simulink model "realtime"  (R2024b)
settings: Solver=ode5  StartTime=0.0  StopTime=45  FixedStep=0.001  RelTol=1e-3
InitFcn:
  | Init
values from neighbouring files (symbols this model uses):
  Beq = 1.223604206496999e-06    (= 1.2236042065e-06)    [DesignPart567.m]    (also in DesignPart9Sine.m; DesignPart9Step.m; Init.m; Real_time_parameter_estimation.m = (data.Beq_hat_pos + data.Beq_hat_neg)/2)
  degs2rpm = 60/360    (= 0.166666666667)    [Init.m]
  delta_est = 1/sqrt(2)    [DesignPart9Step.m]    (also in Init.m)
  Kd = Kp * Td    [Init.m]
  Ki = Kp / Ti    [Init.m]
  Kp = deltak * cos(deltaphi)    [Init.m]
  rpm2degs = 360/60    (= 6)    [Init.m]
  rpm2rads = 2*pi/60    (= 0.10471975512)    [Init.m]
  tau_sf = (abs(data.tau_sf_pos)+abs(data.tau_sf_neg))/2    [Real_time_parameter_estimation.m]    (also in real-time-estimation.mat = 0.0046178193958)
  tl = 1/(3*wgc)    [Init.m]
  wc = 2*pi*50    (= 314.159265359)    [DesignPart9Step.m]    (also in Init.m; State_space_1324.m)
undefined symbols (not defined in the file or in its folder): gbox, mld, mot, National_Instruments, PCI, sens
libraries: sldrtlib x3, simulink x2, SignalEditorBlockLib x1
settings Model: SimulationMode=external  ExtModeTrigDuration=1000001  Creator=galeazzolu  LastModifiedBy=galeazzolu
settings DataIOCC: ReturnWorkspaceOutputs=off
settings HardwareCC: ProdBitPerLong=64  ProdHWDeviceType=Intel->x86-64 (Linux 64)
settings RTWCC: Description=Simulink Desktop Real-Time  SystemTargetFile=sldrt.tlc  TemplateMakefile=sldrt.tmf  RTWCompilerOptimization=on
settings CodeAppCC: MaxIdLength=95
settings SimulinkDesktopRealTimeCC: TargetLibSuffix=_sldrt.a  TargetPreCompLibLocation=C:\Program Files\MATLAB\R2024b\toolbox\sldrt\lib\win64  ParMdlRefBuildCompliant=on

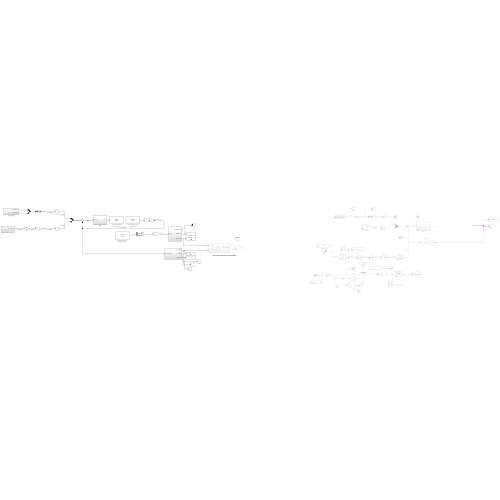
[thumbnail: Simulink's stored preview of the top-level diagram]
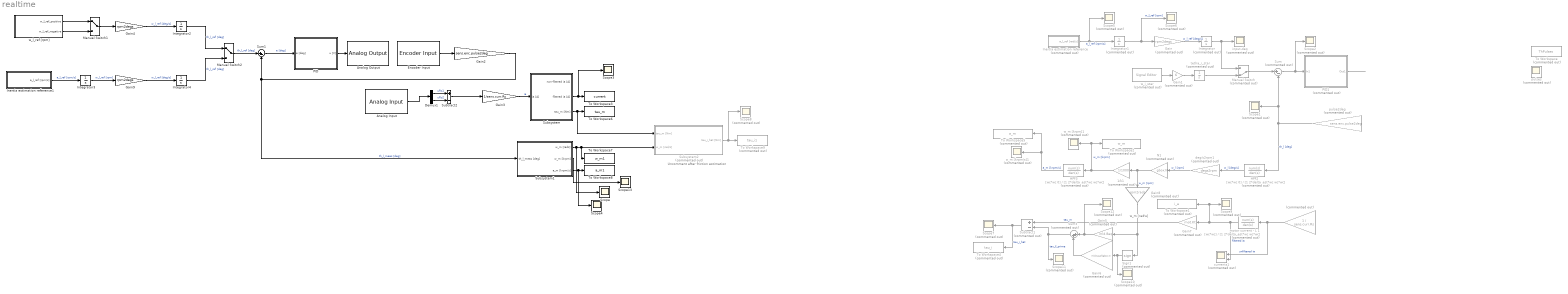
== system realtime ==
  note: w_m [rad\s]
  note: Uncomment after friction estimation
  " " : Gain  Commented=on  Gain=1 / sens.curr.Rs
  1/k1 : Gain  Commented=on  Gain=1/1000
  Analog Input : sldrtlib/Analog Input  SampleTime=-1  MaxMissedTicks=10  ShowMissedTicks=off  YieldWhenWaiting=off  DrvName=National_Instruments/PCI-6221  DrvAddress=4294967295  DrvOptions=[0 0 0 2 0]  Channels=[1,2]  RangeMode=1  VoltRange=1  DataType=1
      settings: AttributesFormatString=National Instruments\nPCI-6221 [auto]
  Analog Output : sldrtlib/Analog Output  SampleTime=-1  MaxMissedTicks=10  ShowMissedTicks=off  YieldWhenWaiting=off  DrvName=National_Instruments/PCI-6221  DrvAddress=4294967295  DrvOptions=[0 0 0 2 0]  Channels=1  RangeMode=1  VoltRange=1  InitialValue=0  FinalValue=0
      settings: AttributesFormatString=National Instruments\nPCI-6221 [auto]
  Demux1 : Demux  Outputs=2
  Encoder Input : sldrtlib/Encoder Input  SampleTime=-1  MaxMissedTicks=10  ShowMissedTicks=off  YieldWhenWaiting=off  DrvName=National_Instruments/PCI-6221  DrvAddress=4294967295  DrvOptions=[0 0 0 2 0]  Channels=1  QuadMode=3  IndexPulse=1  InputFilter=Inf  DataType=1
      settings: AttributesFormatString=National Instruments\nPCI-6221 [auto]
  Gain : Gain  Commented=on  Gain=rpm2degs
  Gain1 : Gain  Commented=on  Gain=6
  Gain2 : Gain  Gain=sens.enc.pulse2deg
  Gain3 : Gain  Gain=1/sens.curr.Rs
  Gain4 : Gain  Gain=rpm2degs
  Gain5 : Gain  Commented=on  Gain=mld.Beq
  Gain6 : Gain  Commented=on  Gain=mld.tausf/gbox.N
  Gain7 : Gain  Commented=on  Gain=mot.Kt
  Gain8 : Gain  Commented=on  Gain=rpm2rads
  Gain9 : Gain  Gain=rpm2degs
  HPF2 : TransferFcn  Commented=on  Numerator=[wc*wc 0]  Denominator=[1 2*delta_est*wc wc*wc]
  HPF3 : TransferFcn  Commented=on  Numerator=[wc*wc 0]  Denominator=[1 2*delta_est*wc wc*wc]
  Inertia estimation reference : Subsystem  Commented=on
  Inertia estimation reference1 : Subsystem
  Integrator : Integrator  Commented=on
  Integrator1 : Integrator  Commented=on
  Integrator2 : Integrator
  Integrator3 : Integrator
  Integrator4 : Integrator
  Manual Switch : ManualSwitch  Commented=on  CurrentSetting=0
  Manual Switch1 : ManualSwitch
  Manual Switch2 : ManualSwitch
  N1 : Gain  Commented=on  Gain=gbox.N
  PID : Subsystem
  PID1 : Subsystem  Commented=on
  Scope{,3..4,13} (4 alike) : Scope
  Scope{1..2,5..12} (10 alike) : Scope  Commented=on
  Sign1 : Signum  Commented=on  ZeroCross=off
  Subsystem : Subsystem
  Subsystem1 : Subsystem
  Subsystem2 : Subsystem  Commented=on
  Subtract1 : Sum  Commented=on  Inputs=+-
  Subtract2 : Sum  Inputs=+-
  Sum : Sum  Commented=on  Inputs=|+-
  Sum1 : Sum  Inputs=|+-
  Sum3 : Sum  Commented=on  Inputs=|++
  To Workspace : ToWorkspace  Commented=on  VariableName=ThPulses  SaveFormat=Structure With Time  SampleTime=-1
  To Workspace1 : ToWorkspace  Commented=on  VariableName=i_a  SaveFormat=Structure With Time  SampleTime=-1
  To Workspace2 : ToWorkspace  Commented=on  VariableName=w_m  SaveFormat=Structure With Time  SampleTime=-1
  To Workspace3 : ToWorkspace  VariableName=current  SaveFormat=Structure With Time  SampleTime=-1
  To Workspace4 : ToWorkspace  Commented=on  VariableName=tau_i  SaveFormat=Structure With Time  SampleTime=-1
  To Workspace5 : ToWorkspace  Commented=on  VariableName=a_m  SaveFormat=Structure With Time  SampleTime=-1
  To Workspace6 : ToWorkspace  VariableName=tau_m  SaveFormat=Structure With Time  SampleTime=-1
  To Workspace7 : ToWorkspace  VariableName=w_m1  SaveFormat=Structure With Time  SampleTime=-1
  To Workspace8 : ToWorkspace  VariableName=a_m1  SaveFormat=Structure With Time  SampleTime=-1
  To Workspace9 : ToWorkspace  Commented=on  VariableName=tau_i1  SaveFormat=Structure With Time  SampleTime=-1
  a_m [krpm/s]1 : Scope  Commented=on
  currents1 : Scope  Commented=on  NumInputPorts=2
  deg/s2rpm1 : Gain  Commented=on  Gain=degs2rpm
  input-deg : Scope  Commented=on
  motor current - L 1 : TransferFcn  Commented=on  Numerator=[wc*wc]  Denominator=[1 2*delta_est*wc wc*wc]
  pulse2deg : Gain  Commented=on  Gain=sens.enc.pulse2deg
  pulses : Scope  Commented=on
  tetha_i_star : Integrator  Commented=on
  w_i_star : SignalEditorBlockLib/Signal Editor  Commented=on  FileName=untitled.mat  ActiveScenario=Scenario  ActiveSignal=Signal 1  IsBus=off  OutputBusObjectStr=Bus: BusObject  SampleTime=0  Interpolate=off  ZeroCross=off  OutputAfterFinalValue=Setting to zero  Unit=inherit  PreserveSignalName=on  ApplySigPropsToAllScenarios=on  ApplySigPropsToAllSignals=off
  w_l_ref [rpm] : Subsystem
  w_m [krpm]1 : Scope  Commented=on
  wires:
  N1/1 -> Gain8/1, 1/k1/1  "w_m [rpm]"
  pulse2deg/1 -> HPF2/1, Sum/2, Scope1/1  "th_l [deg]"
  Sum3/1 -> Subtract1/2, Scope11/1  "tau_f_prime"
  motor current - L 1/1 -> To Workspace1/1, Scope9/1, Gain7/1, currents1/2  "filtered ia"
  Gain/1 -> Integrator/1  "w_l_ref [deg/s]"
  Subtract1/1 -> To Workspace4/1, Scope7/1  "tau_i_hat"
  Gain7/1 -> Subtract1/1  "tau_m"
  HPF2/1 -> deg/s2rpm1/1  "w_l [deg/s]"
  Integrator/1 -> Manual Switch/1, input-deg/1
  ? -> pulses/1, pulse2deg/1, To Workspace/1
  Inertia estimation reference/1(a_l_ref [rad/s]) -> Scope5/1, Integrator1/1  "a_l_ref [rpm/s]"
  Manual Switch/1 -> Sum/1
  Sign1/1 -> Scope10/1, Gain6/1
  deg/s2rpm1/1 -> N1/1  "w_l [rpm]"
  1/k1/1 -> HPF3/1, To Workspace2/1, w_m [krpm]1/1  "w_m [krpm]"
  HPF3/1 -> a_m [krpm/s]1/1, To Workspace5/1  "a_m [krpm/s]"
  PID1/1(Out1) -> ?
  Gain5/1 -> Sum3/1, Scope12/1
  Gain8/1 -> Sign1/1, Gain5/1
  Integrator1/1 -> Scope6/1, Gain/1  "w_l_ref [rpm]"
  Gain6/1 -> Sum3/2
  " "/1 -> currents1/1, motor current - L 1/1  "unfiltered ia"
  Sum/1 -> Scope2/1, PID1/1(In1)
  Gain1/1 -> tetha_i_star/1
  w_i_star/1 -> Gain1/1
  tetha_i_star/1 -> Manual Switch/2
  Subtract2/1 -> Gain3/1
  Manual Switch1/1 -> Gain4/1
  Integrator4/1 -> Manual Switch2/2  "th_l_ref [deg]"
  Inertia estimation reference1/1(a_l_ref [rpm/s]) -> Integrator3/1  "a_l_ref [rpm/s]"
  Encoder Input/1 -> Gain2/1
  Sum1/1 -> PID/1(e [deg])  "e [deg]"
  Gain2/1 -> Subsystem1/1(th_l_meas [deg]), Sum1/2  "th_l_meas [deg]"
  Demux1/2 -> Subtract2/2  "uRs2"
  Gain4/1 -> Integrator2/1  "w_l_ref [deg/s]"
  Gain3/1 -> Subsystem/1(ia [A])  "ia"
  Subsystem2/1(tau_i_hat [Nm]) -> Scope8/1, To Workspace9/1
  w_l_ref [rpm]/1(w_l_ref_positive) -> Manual Switch1/1
  Subsystem/3(tau_m [Nm]) -> Subsystem2/1(tau_m [Nm]), To Workspace6/1
  Integrator2/1 -> Manual Switch2/1  "th_l_ref [deg]"
  Subsystem/2(filtered ia [A]) -> Scope3/1, To Workspace3/1
  Analog Input/1 -> Demux1/1
  Integrator3/1 -> Gain9/1  "w_l_ref [rpm]"
  Subsystem1/1(w_m [rads]) -> Subsystem2/2(w_m [rad/s]), To Workspace7/1, Scope/1
  w_l_ref [rpm]/2(w_l_ref_negative) -> Manual Switch1/2
  PID/1(u [V]) -> Analog Output/1
  Subsystem1/2(w_m [krpm]) -> Scope13/1
  Manual Switch2/1 -> Sum1/1  "th_l_ref [deg]"
  Gain9/1 -> Integrator4/1  "w_l_ref [deg/s]"
  Demux1/1 -> Subtract2/1  "uRs1"
  Subsystem1/3(a_m [krpm/s]) -> Scope4/1, To Workspace8/1

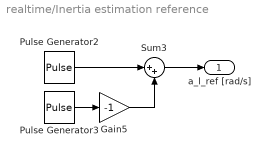
== system realtime/Inertia estimation reference ==
  Gain5 : Gain  Gain=-1
  Pulse Generator2 : DiscretePulseGenerator  PulseType=Time based  Amplitude=450  PulseWidth=50
  Pulse Generator3 : DiscretePulseGenerator  PulseType=Time based  Amplitude=450  PulseWidth=50  PhaseDelay=1
  Sum3 : Sum  Inputs=|++
  a_l_ref [rad/s] : Outport
  wires:
  Pulse Generator3/1 -> Gain5/1
  Pulse Generator2/1 -> Sum3/1
  Gain5/1 -> Sum3/2
  Sum3/1 -> a_l_ref [rad/s]/1

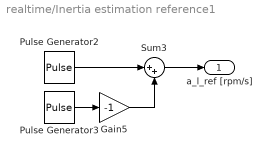
== system realtime/Inertia estimation reference1 ==
  Gain5 : Gain  Gain=-1
  Pulse Generator2 : DiscretePulseGenerator  PulseType=Time based  Amplitude=450  PulseWidth=50
  Pulse Generator3 : DiscretePulseGenerator  PulseType=Time based  Amplitude=450  PulseWidth=50  PhaseDelay=1
  Sum3 : Sum  Inputs=|++
  a_l_ref [rpm/s] : Outport
  wires:
  Pulse Generator3/1 -> Gain5/1
  Pulse Generator2/1 -> Sum3/1
  Gain5/1 -> Sum3/2
  Sum3/1 -> a_l_ref [rpm/s]/1

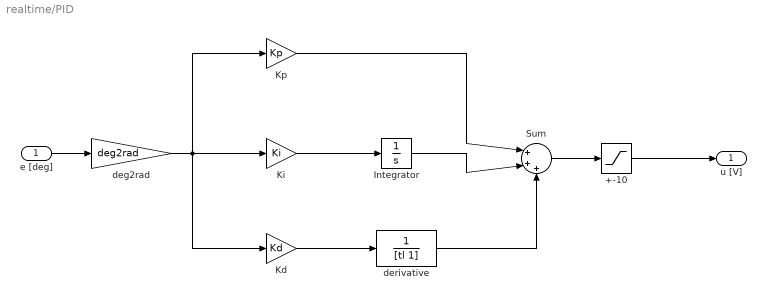
== system realtime/PID ==
  e [deg] : Inport
  +-10 : Saturate  UpperLimit=10  LowerLimit=-10
  Integrator : Integrator
  Kd : Gain  Gain=Kd
  Ki : Gain  Gain=Ki
  Kp : Gain  Gain=Kp
  Sum : Sum  Inputs=|+++
  deg2rad : Gain  Gain=deg2rad
  derivative : TransferFcn  Denominator=[tl 1]
  u [V] : Outport
  wires:
  e [deg]/1 -> deg2rad/1
  deg2rad/1 -> Kd/1, Kp/1, Ki/1
  Ki/1 -> Integrator/1
  Kp/1 -> Sum/1
  Integrator/1 -> Sum/2
  Kd/1 -> derivative/1
  derivative/1 -> Sum/3
  Sum/1 -> +-10/1
  +-10/1 -> u [V]/1

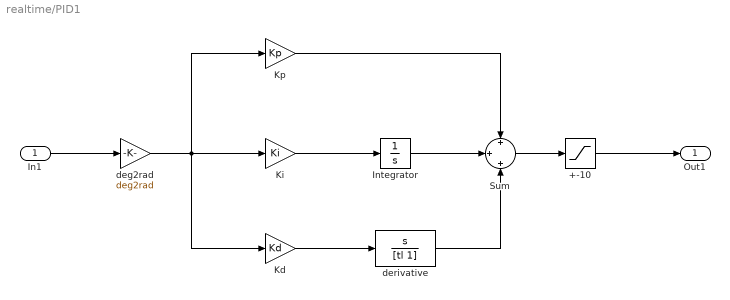
== system realtime/PID1 ==
  In1 : Inport
  +-10 : Saturate  UpperLimit=10  LowerLimit=-10
  Integrator : Integrator
  Kd : Gain  Gain=Kd
  Ki : Gain  Gain=Ki
  Kp : Gain  Gain=Kp
  Sum : Sum  Inputs=+|+|+
  deg2rad : Gain  Gain=deg2rad
  derivative : TransferFcn  Numerator=[1 0]  Denominator=[tl 1]
  Out1 : Outport
  wires:
  In1/1 -> deg2rad/1
  deg2rad/1 -> Kd/1, Kp/1, Ki/1
  Ki/1 -> Integrator/1
  Kp/1 -> Sum/1
  Integrator/1 -> Sum/2
  Kd/1 -> derivative/1
  derivative/1 -> Sum/3
  Sum/1 -> +-10/1
  +-10/1 -> Out1/1

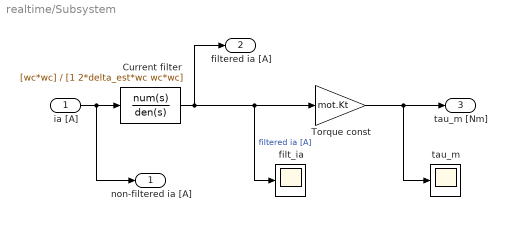
== system realtime/Subsystem ==
  ia [A] : Inport
  " Current filter" : TransferFcn  Numerator=[wc*wc]  Denominator=[1 2*delta_est*wc wc*wc]
  Torque const : Gain  Gain=mot.Kt
  filt_ia : Scope
  tau_m : Scope
  non-filtered ia [A] : Outport
  filtered ia [A] : Outport  Port=2
  tau_m [Nm] : Outport  Port=3
  wires:
  " Current filter"/1 -> filtered ia [A]/1, filt_ia/1, Torque const/1  "filtered ia [A]"
  Torque const/1 -> tau_m [Nm]/1, tau_m/1
  ia [A]/1 -> non-filtered ia [A]/1, " Current filter"/1

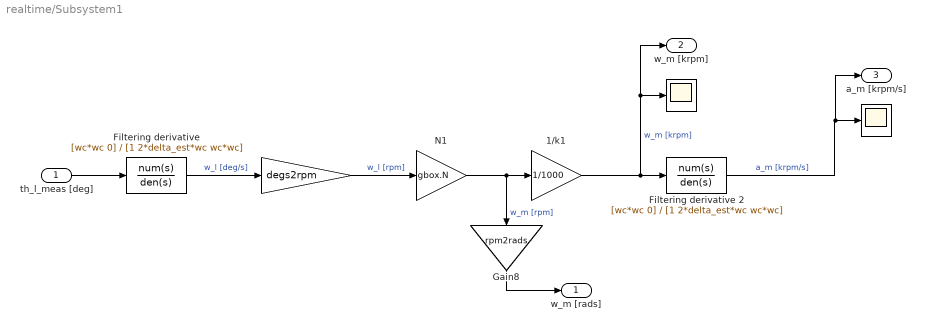
== system realtime/Subsystem1 ==
  th_l_meas [deg] : Inport
  " " : Gain  Gain=degs2rpm
  "  " : Scope
  "    " : Scope
  1/k1 : Gain  Gain=1/1000
  Filtering derivative : TransferFcn  Numerator=[wc*wc 0]  Denominator=[1 2*delta_est*wc wc*wc]
  Filtering derivative 2 : TransferFcn  Numerator=[wc*wc 0]  Denominator=[1 2*delta_est*wc wc*wc]
  Gain8 : Gain  Gain=rpm2rads
  N1 : Gain  Gain=gbox.N
  w_m [rads] : Outport
  w_m [krpm] : Outport  Port=2
  a_m [krpm/s] : Outport  Port=3
  wires:
  N1/1 -> Gain8/1, 1/k1/1  "w_m [rpm]"
  1/k1/1 -> "  "/1, w_m [krpm]/1, Filtering derivative 2/1  "w_m [krpm]"
  Gain8/1 -> w_m [rads]/1
  Filtering derivative/1 -> " "/1  "w_l [deg/s]"
  Filtering derivative 2/1 -> a_m [krpm/s]/1, "    "/1  "a_m [krpm/s]"
  " "/1 -> N1/1  "w_l [rpm]"
  th_l_meas [deg]/1 -> Filtering derivative/1

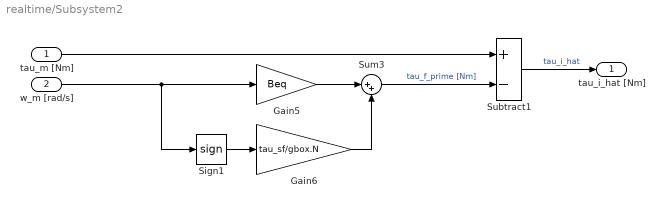
== system realtime/Subsystem2 ==
  tau_m [Nm] : Inport
  w_m [rad/s] : Inport  Port=2
  Gain5 : Gain  Gain=Beq
  Gain6 : Gain  Gain=tau_sf/gbox.N
  Sign1 : Signum  ZeroCross=off
  Subtract1 : Sum  Inputs=+-
  Sum3 : Sum  Inputs=|++
  tau_i_hat [Nm] : Outport
  wires:
  Subtract1/1 -> tau_i_hat [Nm]/1  "tau_i_hat"
  tau_m [Nm]/1 -> Subtract1/1
  Gain5/1 -> Sum3/1
  Sum3/1 -> Subtract1/2  "tau_f_prime [Nm]"
  Sign1/1 -> Gain6/1
  Gain6/1 -> Sum3/2
  w_m [rad/s]/1 -> Sign1/1, Gain5/1

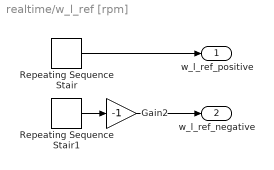
== system realtime/w_l_ref [rpm] ==
  Gain2 : Gain  Gain=-1
  Repeating Sequence Stair : simulink/Sources/Repeating Sequence Stair  OutValues=[50 100 150 200 250 300 350 400 450 450].'  tsamp=5  OutMin=[]  OutMax=[]  OutDataTypeStr=double  OutputDataTypeScalingMode=double  OutDataType=fixdt(0,8)  ConRadixGroup=Best Precision: Vector-wise  OutScaling=2^-12
  Repeating Sequence Stair1 : simulink/Sources/Repeating Sequence Stair  OutValues=[50 100 150 200 250 300 350 400 450 450].'  tsamp=5  OutMin=[]  OutMax=[]  OutDataTypeStr=double  OutputDataTypeScalingMode=double  OutDataType=fixdt(0,8)  ConRadixGroup=Best Precision: Vector-wise  OutScaling=2^-12
  w_l_ref_positive : Outport
  w_l_ref_negative : Outport  Port=2
  wires:
  Repeating Sequence Stair1/1 -> Gain2/1
  Gain2/1 -> w_l_ref_negative/1
  Repeating Sequence Stair/1 -> w_l_ref_positive/1
